simulink model "testing"  (R2019a)
settings: Solver=VariableStepAuto  StartTime=0.0  StopTime=50  RelTol=1e-3
values from neighbouring files (symbols this model uses):
  A = [0 0 0 1 0 0; 0 0 0 0 1 0;0 0 0 0 0 1;0 0 g 0 0 0; 0 0 0 0 0 0; 0 0 0 0 0 0]    [Linearization.m]
  B = [0 0 0;0 0 0;0 0 0;0 1/m g;1/m 0 -g;0 l2/J -m*g*(l1 + ln)/J]    [Linearization.m]
  C = eye(3,6)    [Linearization.m]
  g = 9.81    [Linearization.m]    (also in thrust.m)
  m = 10    [Linearization.m]    (also in thrust.m)
settings Model: Creator=Ankith A Das  LastModifiedBy=Ankith A Das

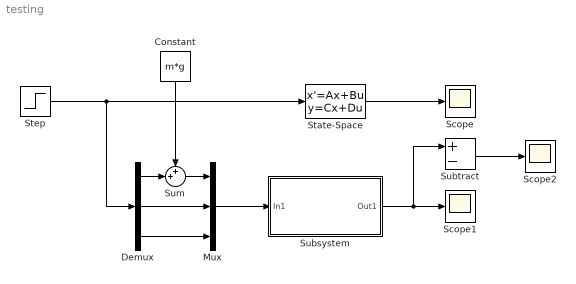
== system testing ==
  Constant : Constant  Value=m*g
  Demux : Demux  Outputs=3
  Mux : Mux  Inputs=3
  Scope : Scope
  Scope1 : Scope
  Scope2 : Scope
  State-Space : StateSpace  A=A  B=B  C=C  D=zeros(3,3)  InitialCondition=0
  Step : Step  Time=0  After=[m*g,0,0]'  SampleTime=0
  Subsystem : Subsystem
  Subtract : Sum  Inputs=+-
  Sum : Sum  Inputs=++|
  wires:
  Step/1 -> State-Space/1, Demux/1
  Subsystem/1(Out1) -> Subtract/1, Scope1/1
  Demux/1 -> Sum/2
  Constant/1 -> Sum/1
  Demux/3 -> Mux/3
  Demux/2 -> Mux/2
  Sum/1 -> Mux/1
  Mux/1 -> Subsystem/1(In1)
  Subtract/1 -> Scope2/1
  State-Space/1 -> Scope/1

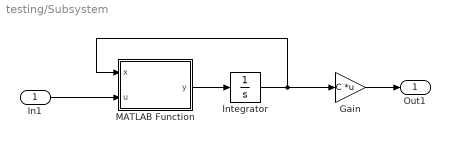
== system testing/Subsystem ==
  In1 : Inport
  Gain : Gain  Gain=C  Multiplication=Matrix(K*u)
  Integrator : Integrator  InitialCondition=[0,0,0,0,0,0]
  MATLAB Function : MATLAB Function  TreatAsAtomicUnit=on
  Out1 : Outport
  wires:
  In1/1 -> MATLAB Function/2(u)
  Integrator/1 -> Gain/1, MATLAB Function/1(x)
  MATLAB Function/1(y) -> Integrator/1
  Gain/1 -> Out1/1

== matlab function testing/Subsystem/MATLAB Function ==
  data: x input; u input; y output
function y = fcn(x,u)
    y = thrust(x,u);
